simulink model "Alireza_3P_FuzzyPID"  (R2023a)
settings: Solver=VariableStepAuto  StartTime=0.0  StopTime=4  RelTol=1e-3
libraries: fuzblock x3, slpidlib x3
settings Model: Creator=Javad  LastModifiedBy=Alireza
settings SolverCC: AlgebraicLoopSolver=TrustRegion
settings DebuggingCC: UnconnectedInputMsg=warning  UnconnectedOutputMsg=warning  UnconnectedLineMsg=warning
settings ModelReferenceCC: EnableRefExpFcnMdlSchedulingChecks=on

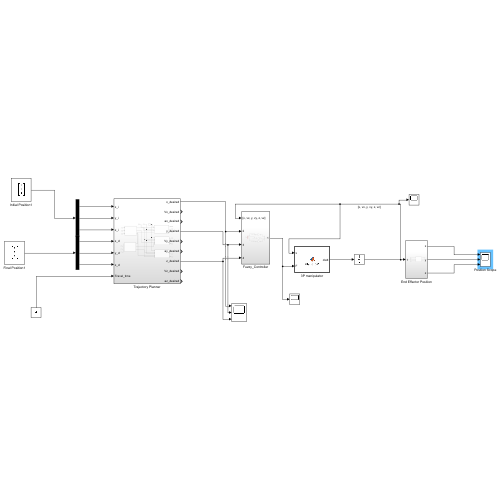
[thumbnail: Simulink's stored preview of the top-level diagram]
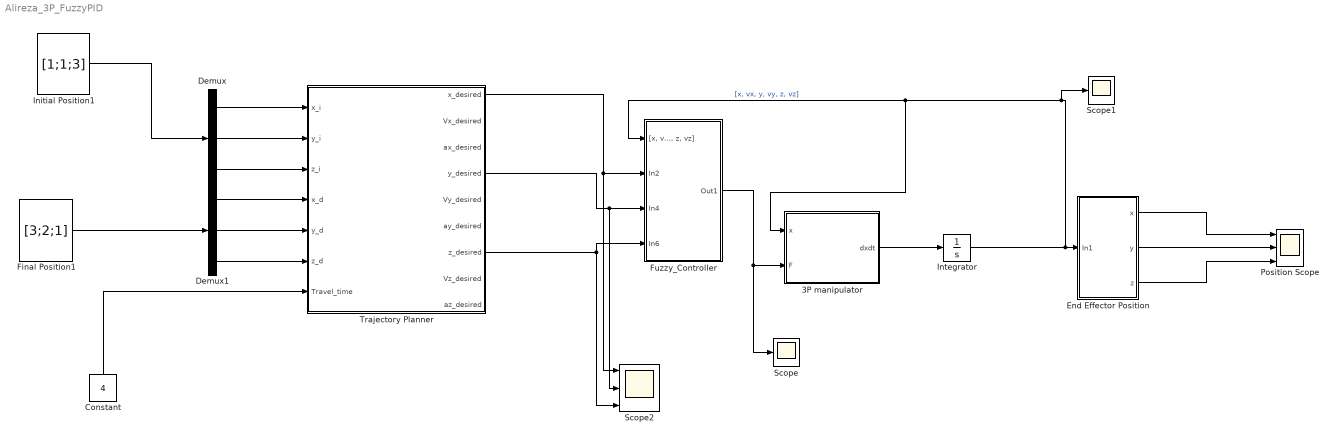
== system Alireza_3P_FuzzyPID ==
  3P manipulator : MATLAB Function  TreatAsAtomicUnit=on
  Constant : Constant  Value=4
  Demux : Demux  Outputs=3
  Demux1 : Demux  Outputs=3
  End Effector Position : Subsystem
  Final Position1 : Constant  Value=[3;2;1]  VectorParams1D=off
  Fuzzy_Controller : Subsystem
  Initial Position1 : Constant  Value=[1;1;3]  VectorParams1D=off
  Integrator : Integrator  InitialCondition=[0.5;0; 0.5;0; 2.8;0]
  Position Scope : Scope  NumInputPorts=3
  Scope : Scope
  Scope1 : Scope
  Scope2 : Scope  NumInputPorts=3
  Trajectory Planner : Subsystem
  wires:
  Demux/1 -> Trajectory Planner/1(x_i)
  Demux/2 -> Trajectory Planner/2(y_i)
  Demux/3 -> Trajectory Planner/3(z_i)
  Demux1/1 -> Trajectory Planner/4(x_d)
  Demux1/2 -> Trajectory Planner/5(y_d)
  Demux1/3 -> Trajectory Planner/6(z_d)
  3P manipulator/1(dxdt) -> Integrator/1
  Integrator/1 -> Scope1/1, 3P manipulator/1(x), Fuzzy_Controller/1("[x, vx, y, vy, z, vz]"), End Effector Position/1(In1)  "[x, vx, y, vy, z, vz]"
  End Effector Position/1(x) -> Position Scope/1
  End Effector Position/2(y) -> Position Scope/2
  End Effector Position/3(z) -> Position Scope/3
  Trajectory Planner/1(x_desired) -> Fuzzy_Controller/2(In2), Scope2/1
  Trajectory Planner/4(y_desired) -> Scope2/2, Fuzzy_Controller/3(In4)
  Trajectory Planner/7(z_desired) -> Fuzzy_Controller/4(In6), Scope2/3
  Fuzzy_Controller/1(Out1) -> Scope/1, 3P manipulator/2(F)
  Initial Position1/1 -> Demux/1
  Final Position1/1 -> Demux1/1
  Constant/1 -> Trajectory Planner/7(Travel_time)

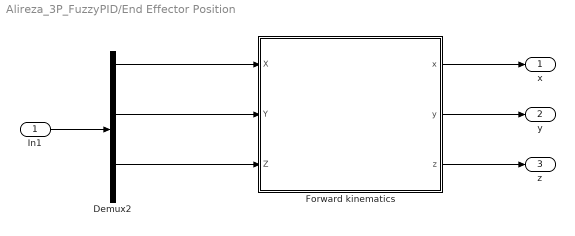
== system Alireza_3P_FuzzyPID/End Effector Position ==
  In1 : Inport
  Demux2 : Demux  Outputs=6
  Forward kinematics : MATLAB Function  TreatAsAtomicUnit=on
  x : Outport
  y : Outport  Port=2
  z : Outport  Port=3
  wires:
  Demux2/1 -> Forward kinematics/1(X)
  In1/1 -> Demux2/1
  Forward kinematics/2(y) -> y/1
  Demux2/3 -> Forward kinematics/2(Y)
  Forward kinematics/3(z) -> z/1
  Forward kinematics/1(x) -> x/1
  Demux2/5 -> Forward kinematics/3(Z)

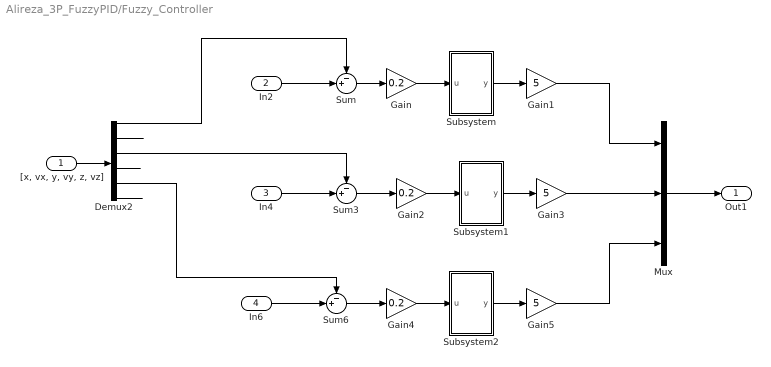
== system Alireza_3P_FuzzyPID/Fuzzy_Controller ==
  "[x, vx, y, vy, z, vz]" : Inport
  In2 : Inport  Port=2
  In4 : Inport  Port=3
  In6 : Inport  Port=4
  Demux2 : Demux  Outputs=6
  Gain : Gain  Gain=0.2
  Gain1 : Gain  Gain=5
  Gain2 : Gain  Gain=0.2
  Gain3 : Gain  Gain=5
  Gain4 : Gain  Gain=0.2
  Gain5 : Gain  Gain=5
  Mux : Mux  Inputs=3
  Subsystem : Subsystem
  Subsystem1 : Subsystem
  Subsystem2 : Subsystem
  Sum : Sum  Inputs=-+|
  Sum3 : Sum  Inputs=-+|
  Sum6 : Sum  Inputs=-+|
  Out1 : Outport
  wires:
  In2/1 -> Sum/2
  Demux2/5 -> Sum6/1
  In4/1 -> Sum3/2
  Demux2/1 -> Sum/1
  Demux2/2 -> ?
  Demux2/3 -> Sum3/1
  Mux/1 -> Out1/1
  In6/1 -> Sum6/2
  Demux2/4 -> ?
  Demux2/6 -> ?
  "[x, vx, y, vy, z, vz]"/1 -> Demux2/1
  Sum/1 -> Gain/1
  Gain/1 -> Subsystem/1(u)
  Subsystem/1(y) -> Gain1/1
  Gain1/1 -> Mux/1
  Subsystem1/1(y) -> Gain3/1
  Gain2/1 -> Subsystem1/1(u)
  Sum3/1 -> Gain2/1
  Gain3/1 -> Mux/2
  Gain5/1 -> Mux/3
  Gain4/1 -> Subsystem2/1(u)
  Subsystem2/1(y) -> Gain5/1
  Sum6/1 -> Gain4/1

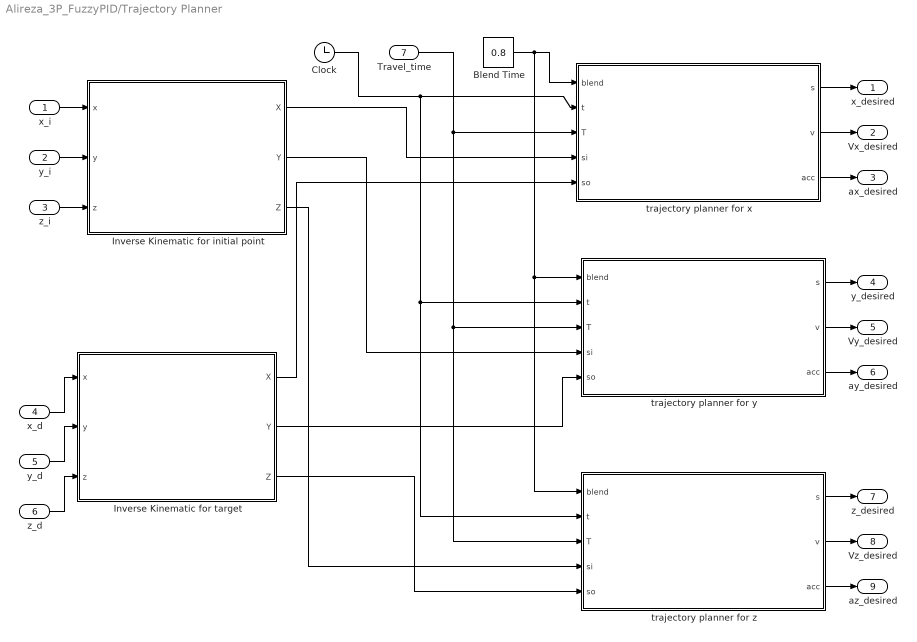
== system Alireza_3P_FuzzyPID/Trajectory Planner ==
  x_i : Inport
  y_i : Inport  Port=2
  z_i : Inport  Port=3
  x_d : Inport  Port=4
  y_d : Inport  Port=5
  z_d : Inport  Port=6
  Travel_time : Inport  Port=7
  Blend Time : Constant  Value=0.8
  Clock : Clock
  Inverse Kinematic for initial point : MATLAB Function  TreatAsAtomicUnit=on
  Inverse Kinematic for target : MATLAB Function  TreatAsAtomicUnit=on
  trajectory planner for x : MATLAB Function  TreatAsAtomicUnit=on
  trajectory planner for y : MATLAB Function  TreatAsAtomicUnit=on
  trajectory planner for z : MATLAB Function  TreatAsAtomicUnit=on
  x_desired : Outport
  Vx_desired : Outport  Port=2
  ax_desired : Outport  Port=3
  y_desired : Outport  Port=4
  Vy_desired : Outport  Port=5
  ay_desired : Outport  Port=6
  z_desired : Outport  Port=7
  Vz_desired : Outport  Port=8
  az_desired : Outport  Port=9
  wires:
  trajectory planner for x/2(v) -> Vx_desired/1
  y_i/1 -> Inverse Kinematic for initial point/2(y)
  trajectory planner for x/1(s) -> x_desired/1
  Inverse Kinematic for initial point/1(X) -> trajectory planner for x/4(si)
  Inverse Kinematic for target/1(X) -> trajectory planner for x/5(so)
  trajectory planner for x/3(acc) -> ax_desired/1
  x_i/1 -> Inverse Kinematic for initial point/1(x)
  z_i/1 -> Inverse Kinematic for initial point/3(z)
  Inverse Kinematic for initial point/2(Y) -> trajectory planner for y/4(si)
  trajectory planner for y/3(acc) -> ay_desired/1
  trajectory planner for y/2(v) -> Vy_desired/1
  trajectory planner for y/1(s) -> y_desired/1
  Inverse Kinematic for target/2(Y) -> trajectory planner for y/5(so)
  Clock/1 -> trajectory planner for x/2(t), trajectory planner for z/2(t), trajectory planner for y/2(t)
  Inverse Kinematic for target/3(Z) -> trajectory planner for z/5(so)
  trajectory planner for z/1(s) -> z_desired/1
  Inverse Kinematic for initial point/3(Z) -> trajectory planner for z/4(si)
  Travel_time/1 -> trajectory planner for x/3(T), trajectory planner for y/3(T), trajectory planner for z/3(T)
  trajectory planner for z/2(v) -> Vz_desired/1
  Blend Time/1 -> trajectory planner for y/1(blend), trajectory planner for z/1(blend), trajectory planner for x/1(blend)
  trajectory planner for z/3(acc) -> az_desired/1
  z_d/1 -> Inverse Kinematic for target/3(z)
  x_d/1 -> Inverse Kinematic for target/1(x)
  y_d/1 -> Inverse Kinematic for target/2(y)

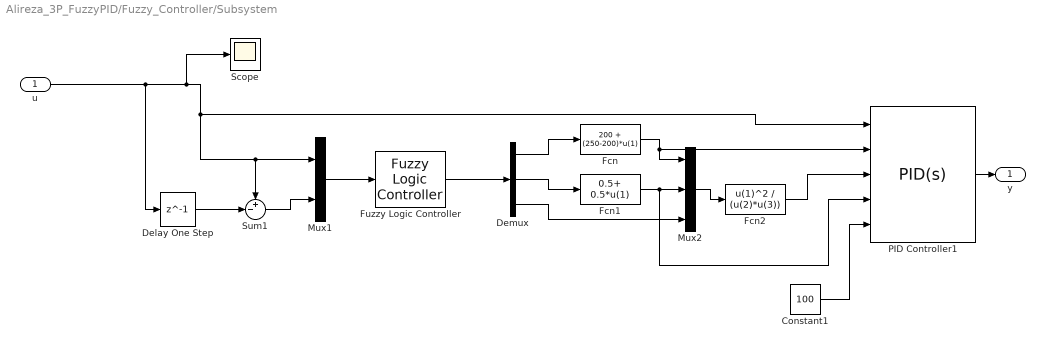
== system Alireza_3P_FuzzyPID/Fuzzy_Controller/Subsystem ==
  u : Inport
  Constant1 : Constant  Value=100
  Delay One Step : Delay  DelayLength=1
  Demux : Demux  Outputs=3
  Fcn : Fcn  Expr=200 + (250-200)*u(1)
  Fcn1 : Fcn  Expr=0.5+ 0.5*u(1)
  Fcn2 : Fcn  Expr=u(1)^2 / (u(2)*u(3))
  Fuzzy Logic Controller : fuzblock/Fuzzy Logic  Controller  FIS=fuzzy2  OutputSampleNumber=101  DataType=double  FuzzifiedInputs=off  RuleFiringStrengths=off  RuleOutputs=off  AggregatedOutputs=off  SimulateUsing=Code generation  OutOfRangeInputValueMessage=warning  NoRuleFiredMessage=warning  EmptyOutputFuzzySetMessage=warning
  Mux1 : Mux  Inputs=2
  Mux2 : Mux  Inputs=3
  PID Controller1 : slpidlib/PID Controller  Controller=PID  Form=Parallel  TimeDomain=Continuous-time  UseExternalTs=off  SampleTime=-1  IntegratorMethod=Forward Euler  FilterMethod=Forward Euler  ControllerParametersSource=external  P=4.74196748645127  I=1  UseKiTs=off  D=0  N=100  UseFilter=on  TunerSelectOption=Transfer Function Based (PID Tuner App)  InitialConditionSource=internal  InitialConditionForIntegrator=0  InitialConditionForFilter=0  DifferentiatorICPrevScaledInput=0  ExternalReset=none  TrackingMode=off  Kt=1  LimitOutput=off  SatLimitsSource=internal  UpperSaturationLimit=inf  LowerSaturationLimit=-inf  LinearizeAsGain=on  AntiWindupMode=none  Kb=1  LimitIntegrator=off  UpperIntegratorSaturationLimit=inf  LowerIntegratorSaturationLimit=-inf  POutMin=[]  POutMax=[]  IOutMin=[]  IOutMax=[]  DOutMin=[]  DOutMax=[]  NOutMin=[]  NOutMax=[]  SumOutMin=[]  SumOutMax=[]  SaturationOutMin=[]  SaturationOutMax=[]  PParamMin=[]  PParamMax=[]  IParamMin=[]  IParamMax=[]  DParamMin=[]  DParamMax=[]  NParamMin=[]  NParamMax=[]  KbParamMin=[]  KbParamMax=[]  KtParamMin=[]  KtParamMax=[]  KbOutMin=[]  KbOutMax=[]  KtOutMin=[]  KtOutMax=[]  IntegratorOutMin=[]  IntegratorOutMax=[]  FilterOutMin=[]  FilterOutMax=[]  SumI1OutMin=[]  SumI1OutMax=[]  SumI2OutMin=[]  SumI2OutMax=[]  SumI3OutMin=[]  SumI3OutMax=[]  SumI4OutMin=[]  SumI4OutMax=[]  SumDOutMin=[]  SumDOutMax=[]  DifferentiatorOutMin=[]  DifferentiatorOutMax=[]  FilterDiffOutCoefMin=[]  FilterDiffOutCoefMax=[]  ReciprocalOutMin=[]  ReciprocalOutMax=[]  SumDenOutMin=[]  SumDenOutMax=[]  SumNumOutMin=[]  SumNumOutMax=[]  DivideOutMin=[]  DivideOutMax=[]  UdiffTsProdOutMin=[]  UdiffTsProdOutMax=[]  NTsProdOutMin=[]  NTsProdOutMax=[]  UintegralTsProdOutMin=[]  UintegralTsProdOutMax=[]  UngainTsProdOutMin=[]  UngainTsProdOutMax=[]  ClampingZeroOutDataTypeStr=Inherit: Inherit via back propagation  ClampingZeroOutMin=[]  ClampingZeroOutMax=[]  FilterDenConstantOutDataTypeStr=Inherit: Inherit via back propagation  FilterDenConstantOutMin=[]  FilterDenConstantOutMax=[]  PCopyOutDataTypeStr=Inherit: Inherit via back propagation  PCopyOutMin=[]  PCopyOutMax=[]  NCopyOutDataTypeStr=Inherit: Inherit via back propagation  NCopyOutMin=[]  NCopyOutMax=[]  IntegratorContinuousStateAttributes=''  IntegratorStateMustResolveToSignalObject=off  IntegratorRTWStateStorageClass=Auto  FilterContinuousStateAttributes=''  FilterStateMustResolveToSignalObject=off  FilterRTWStateStorageClass=Auto  ParallelPVariant=ExternalParameters  IdealPVariant=Disabled  IVariant=ExternalParameters  DVariant=ExternalParameters  IntegratorVariant=Continuous  SatVariant=Disabled  AWVariant=Passthrough  PCopyVariant=Disabled  TRVariant=Disabled  FdbkBlocksVariant=Forward  IdealPFdbkVariant=Disabled  SatFdbkVariant=Disabled  DerivativeFilterVariant=ContFilter  NVariant=ExternalParameters  NCopyVariant=Disabled  FilterICVariant=InternalICsFilter  IntegratorICVariant=InternalICs  ExternalResetVariant=Disabled  TRSumVariant=Passthrough  SumFdbkVariant=Disabled  SumVariant=Sum_PID  TsampFilterVariant=InternalTs  TsampNgainVariant=Passthrough  TsampIntegralVariant=Disabled_SignalSpec  ExternalSaturationOutDataTypeStr=Inherit: Same as second input
  Scope : Scope
  Sum1 : Sum  Inputs=+-|
  y : Outport
  wires:
  Demux/1 -> Fcn/1
  Constant1/1 -> PID Controller1/5
  Mux1/1 -> Fuzzy Logic Controller/1
  Fuzzy Logic Controller/1 -> Demux/1
  Fcn/1 -> Mux2/1, PID Controller1/2
  Sum1/1 -> Mux1/2
  Delay One Step/1 -> Sum1/2
  Fcn2/1 -> PID Controller1/3
  Fcn1/1 -> PID Controller1/4, Mux2/2
  Mux2/1 -> Fcn2/1
  u/1 -> Delay One Step/1, Scope/1, Sum1/1, Mux1/1, PID Controller1/1
  Demux/2 -> Fcn1/1
  PID Controller1/1 -> y/1
  Demux/3 -> Mux2/3

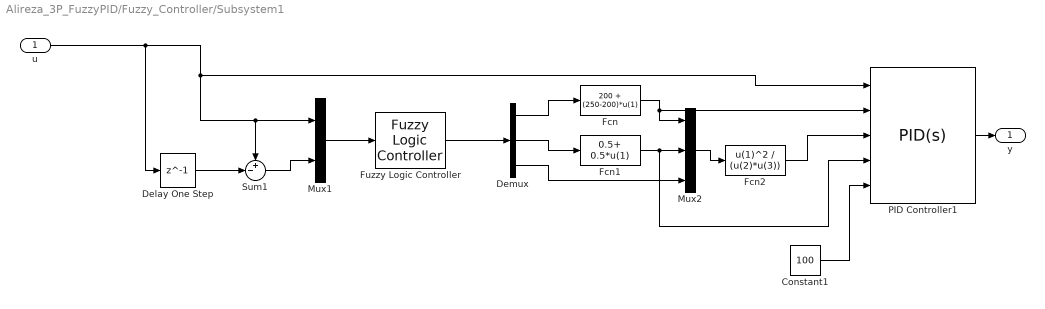
== system Alireza_3P_FuzzyPID/Fuzzy_Controller/Subsystem1 ==
  u : Inport
  Constant1 : Constant  Value=100
  Delay One Step : Delay  DelayLength=1
  Demux : Demux  Outputs=3
  Fcn : Fcn  Expr=200 + (250-200)*u(1)
  Fcn1 : Fcn  Expr=0.5+ 0.5*u(1)
  Fcn2 : Fcn  Expr=u(1)^2 / (u(2)*u(3))
  Fuzzy Logic Controller : fuzblock/Fuzzy Logic  Controller  FIS=fuzzy2  OutputSampleNumber=101  DataType=double  FuzzifiedInputs=off  RuleFiringStrengths=off  RuleOutputs=off  AggregatedOutputs=off  SimulateUsing=Code generation  OutOfRangeInputValueMessage=warning  NoRuleFiredMessage=warning  EmptyOutputFuzzySetMessage=warning
  Mux1 : Mux  Inputs=2
  Mux2 : Mux  Inputs=3
  PID Controller1 : slpidlib/PID Controller  Controller=PID  Form=Parallel  TimeDomain=Continuous-time  UseExternalTs=off  SampleTime=-1  IntegratorMethod=Forward Euler  FilterMethod=Forward Euler  ControllerParametersSource=external  P=4.74196748645127  I=1  UseKiTs=off  D=0  N=100  UseFilter=on  TunerSelectOption=Transfer Function Based (PID Tuner App)  InitialConditionSource=internal  InitialConditionForIntegrator=0  InitialConditionForFilter=0  DifferentiatorICPrevScaledInput=0  ExternalReset=none  TrackingMode=off  Kt=1  LimitOutput=off  SatLimitsSource=internal  UpperSaturationLimit=inf  LowerSaturationLimit=-inf  LinearizeAsGain=on  AntiWindupMode=none  Kb=1  LimitIntegrator=off  UpperIntegratorSaturationLimit=inf  LowerIntegratorSaturationLimit=-inf  POutMin=[]  POutMax=[]  IOutMin=[]  IOutMax=[]  DOutMin=[]  DOutMax=[]  NOutMin=[]  NOutMax=[]  SumOutMin=[]  SumOutMax=[]  SaturationOutMin=[]  SaturationOutMax=[]  PParamMin=[]  PParamMax=[]  IParamMin=[]  IParamMax=[]  DParamMin=[]  DParamMax=[]  NParamMin=[]  NParamMax=[]  KbParamMin=[]  KbParamMax=[]  KtParamMin=[]  KtParamMax=[]  KbOutMin=[]  KbOutMax=[]  KtOutMin=[]  KtOutMax=[]  IntegratorOutMin=[]  IntegratorOutMax=[]  FilterOutMin=[]  FilterOutMax=[]  SumI1OutMin=[]  SumI1OutMax=[]  SumI2OutMin=[]  SumI2OutMax=[]  SumI3OutMin=[]  SumI3OutMax=[]  SumI4OutMin=[]  SumI4OutMax=[]  SumDOutMin=[]  SumDOutMax=[]  DifferentiatorOutMin=[]  DifferentiatorOutMax=[]  FilterDiffOutCoefMin=[]  FilterDiffOutCoefMax=[]  ReciprocalOutMin=[]  ReciprocalOutMax=[]  SumDenOutMin=[]  SumDenOutMax=[]  SumNumOutMin=[]  SumNumOutMax=[]  DivideOutMin=[]  DivideOutMax=[]  UdiffTsProdOutMin=[]  UdiffTsProdOutMax=[]  NTsProdOutMin=[]  NTsProdOutMax=[]  UintegralTsProdOutMin=[]  UintegralTsProdOutMax=[]  UngainTsProdOutMin=[]  UngainTsProdOutMax=[]  ClampingZeroOutDataTypeStr=Inherit: Inherit via back propagation  ClampingZeroOutMin=[]  ClampingZeroOutMax=[]  FilterDenConstantOutDataTypeStr=Inherit: Inherit via back propagation  FilterDenConstantOutMin=[]  FilterDenConstantOutMax=[]  PCopyOutDataTypeStr=Inherit: Inherit via back propagation  PCopyOutMin=[]  PCopyOutMax=[]  NCopyOutDataTypeStr=Inherit: Inherit via back propagation  NCopyOutMin=[]  NCopyOutMax=[]  IntegratorContinuousStateAttributes=''  IntegratorStateMustResolveToSignalObject=off  IntegratorRTWStateStorageClass=Auto  FilterContinuousStateAttributes=''  FilterStateMustResolveToSignalObject=off  FilterRTWStateStorageClass=Auto  ParallelPVariant=ExternalParameters  IdealPVariant=Disabled  IVariant=ExternalParameters  DVariant=ExternalParameters  IntegratorVariant=Continuous  SatVariant=Disabled  AWVariant=Passthrough  PCopyVariant=Disabled  TRVariant=Disabled  FdbkBlocksVariant=Forward  IdealPFdbkVariant=Disabled  SatFdbkVariant=Disabled  DerivativeFilterVariant=ContFilter  NVariant=ExternalParameters  NCopyVariant=Disabled  FilterICVariant=InternalICsFilter  IntegratorICVariant=InternalICs  ExternalResetVariant=Disabled  TRSumVariant=Passthrough  SumFdbkVariant=Disabled  SumVariant=Sum_PID  TsampFilterVariant=InternalTs  TsampNgainVariant=Passthrough  TsampIntegralVariant=Disabled_SignalSpec  ExternalSaturationOutDataTypeStr=Inherit: Same as second input
  Sum1 : Sum  Inputs=+-|
  y : Outport
  wires:
  Demux/3 -> Mux2/3
  PID Controller1/1 -> y/1
  Demux/2 -> Fcn1/1
  u/1 -> PID Controller1/1, Mux1/1, Sum1/1, Delay One Step/1
  Mux2/1 -> Fcn2/1
  Fcn1/1 -> Mux2/2, PID Controller1/4
  Fcn2/1 -> PID Controller1/3
  Delay One Step/1 -> Sum1/2
  Sum1/1 -> Mux1/2
  Fcn/1 -> PID Controller1/2, Mux2/1
  Fuzzy Logic Controller/1 -> Demux/1
  Mux1/1 -> Fuzzy Logic Controller/1
  Constant1/1 -> PID Controller1/5
  Demux/1 -> Fcn/1

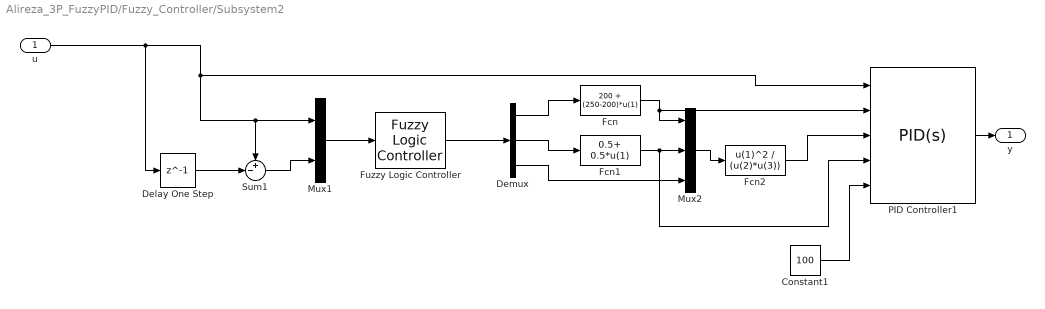
== system Alireza_3P_FuzzyPID/Fuzzy_Controller/Subsystem2 ==
  u : Inport
  Constant1 : Constant  Value=100
  Delay One Step : Delay  DelayLength=1
  Demux : Demux  Outputs=3
  Fcn : Fcn  Expr=200 + (250-200)*u(1)
  Fcn1 : Fcn  Expr=0.5+ 0.5*u(1)
  Fcn2 : Fcn  Expr=u(1)^2 / (u(2)*u(3))
  Fuzzy Logic Controller : fuzblock/Fuzzy Logic  Controller  FIS=fuzzy2  OutputSampleNumber=101  DataType=double  FuzzifiedInputs=off  RuleFiringStrengths=off  RuleOutputs=off  AggregatedOutputs=off  SimulateUsing=Code generation  OutOfRangeInputValueMessage=warning  NoRuleFiredMessage=warning  EmptyOutputFuzzySetMessage=warning
  Mux1 : Mux  Inputs=2
  Mux2 : Mux  Inputs=3
  PID Controller1 : slpidlib/PID Controller  Controller=PID  Form=Parallel  TimeDomain=Continuous-time  UseExternalTs=off  SampleTime=-1  IntegratorMethod=Forward Euler  FilterMethod=Forward Euler  ControllerParametersSource=external  P=4.74196748645127  I=1  UseKiTs=off  D=0  N=100  UseFilter=on  TunerSelectOption=Transfer Function Based (PID Tuner App)  InitialConditionSource=internal  InitialConditionForIntegrator=0  InitialConditionForFilter=0  DifferentiatorICPrevScaledInput=0  ExternalReset=none  TrackingMode=off  Kt=1  LimitOutput=off  SatLimitsSource=internal  UpperSaturationLimit=inf  LowerSaturationLimit=-inf  LinearizeAsGain=on  AntiWindupMode=none  Kb=1  LimitIntegrator=off  UpperIntegratorSaturationLimit=inf  LowerIntegratorSaturationLimit=-inf  POutMin=[]  POutMax=[]  IOutMin=[]  IOutMax=[]  DOutMin=[]  DOutMax=[]  NOutMin=[]  NOutMax=[]  SumOutMin=[]  SumOutMax=[]  SaturationOutMin=[]  SaturationOutMax=[]  PParamMin=[]  PParamMax=[]  IParamMin=[]  IParamMax=[]  DParamMin=[]  DParamMax=[]  NParamMin=[]  NParamMax=[]  KbParamMin=[]  KbParamMax=[]  KtParamMin=[]  KtParamMax=[]  KbOutMin=[]  KbOutMax=[]  KtOutMin=[]  KtOutMax=[]  IntegratorOutMin=[]  IntegratorOutMax=[]  FilterOutMin=[]  FilterOutMax=[]  SumI1OutMin=[]  SumI1OutMax=[]  SumI2OutMin=[]  SumI2OutMax=[]  SumI3OutMin=[]  SumI3OutMax=[]  SumI4OutMin=[]  SumI4OutMax=[]  SumDOutMin=[]  SumDOutMax=[]  DifferentiatorOutMin=[]  DifferentiatorOutMax=[]  FilterDiffOutCoefMin=[]  FilterDiffOutCoefMax=[]  ReciprocalOutMin=[]  ReciprocalOutMax=[]  SumDenOutMin=[]  SumDenOutMax=[]  SumNumOutMin=[]  SumNumOutMax=[]  DivideOutMin=[]  DivideOutMax=[]  UdiffTsProdOutMin=[]  UdiffTsProdOutMax=[]  NTsProdOutMin=[]  NTsProdOutMax=[]  UintegralTsProdOutMin=[]  UintegralTsProdOutMax=[]  UngainTsProdOutMin=[]  UngainTsProdOutMax=[]  ClampingZeroOutDataTypeStr=Inherit: Inherit via back propagation  ClampingZeroOutMin=[]  ClampingZeroOutMax=[]  FilterDenConstantOutDataTypeStr=Inherit: Inherit via back propagation  FilterDenConstantOutMin=[]  FilterDenConstantOutMax=[]  PCopyOutDataTypeStr=Inherit: Inherit via back propagation  PCopyOutMin=[]  PCopyOutMax=[]  NCopyOutDataTypeStr=Inherit: Inherit via back propagation  NCopyOutMin=[]  NCopyOutMax=[]  IntegratorContinuousStateAttributes=''  IntegratorStateMustResolveToSignalObject=off  IntegratorRTWStateStorageClass=Auto  FilterContinuousStateAttributes=''  FilterStateMustResolveToSignalObject=off  FilterRTWStateStorageClass=Auto  ParallelPVariant=ExternalParameters  IdealPVariant=Disabled  IVariant=ExternalParameters  DVariant=ExternalParameters  IntegratorVariant=Continuous  SatVariant=Disabled  AWVariant=Passthrough  PCopyVariant=Disabled  TRVariant=Disabled  FdbkBlocksVariant=Forward  IdealPFdbkVariant=Disabled  SatFdbkVariant=Disabled  DerivativeFilterVariant=ContFilter  NVariant=ExternalParameters  NCopyVariant=Disabled  FilterICVariant=InternalICsFilter  IntegratorICVariant=InternalICs  ExternalResetVariant=Disabled  TRSumVariant=Passthrough  SumFdbkVariant=Disabled  SumVariant=Sum_PID  TsampFilterVariant=InternalTs  TsampNgainVariant=Passthrough  TsampIntegralVariant=Disabled_SignalSpec  ExternalSaturationOutDataTypeStr=Inherit: Same as second input
  Sum1 : Sum  Inputs=+-|
  y : Outport
  wires:
  Demux/1 -> Fcn/1
  Constant1/1 -> PID Controller1/5
  Mux1/1 -> Fuzzy Logic Controller/1
  Fuzzy Logic Controller/1 -> Demux/1
  Fcn/1 -> Mux2/1, PID Controller1/2
  Sum1/1 -> Mux1/2
  Delay One Step/1 -> Sum1/2
  Fcn2/1 -> PID Controller1/3
  Fcn1/1 -> PID Controller1/4, Mux2/2
  Mux2/1 -> Fcn2/1
  u/1 -> Delay One Step/1, Sum1/1, Mux1/1, PID Controller1/1
  Demux/2 -> Fcn1/1
  PID Controller1/1 -> y/1
  Demux/3 -> Mux2/3

== matlab function Alireza_3P_FuzzyPID/Trajectory Planner/Inverse Kinematic for initial point ==
  data: x input; X output; y input; z input; Y output; Z output
function [X, Y, Z] = inverse_kinematic(x, y, z)

L1=0.5; L2=0.5; L3=0.2;
X=x-L1;
Y=y-L2;
Z=z-L3;

end

== matlab function Alireza_3P_FuzzyPID/3P manipulator ==
  data: x input size=[6,1]; dxdt output size=[6,1]; F input size=[3,1]

function dxdt = Plant_3P (x, F)
m1 = 15; m2 = 10; m3 = 5; M =1; g=9.8;
dxdt = zeros(6,1);
dxdt(1) = x(2);
dxdt(2) = 1/(m2+m3+M)*(F(1));
dxdt(3) = x(4);
dxdt(4) = 1/(m1+m2+m3+M)*(F(2));
dxdt(5) = x(6);
dxdt(6) = 1/(M+m3)*(-(M+m3)*g+F(3));

end

== matlab function Alireza_3P_FuzzyPID/Trajectory Planner/trajectory planner for x ==
  data: blend input; t input; s output; T input; si input; so input; v output; acc output
function [s, v, acc] = trajectory_planner(blend, t, T, si, so)
%t is the current time
%T is the toal time of the movement. 
%si is the initial position
%so is the target position
% blend = 1;

V_max = (so-si)/(T-blend);
a = V_max/blend;

if t<=blend
    acc = a;
    v = a*t;
    s = 1/2*a*t.^2+si;
elseif t<=(T-blend)
    acc = 0;
    v = V_max;
    s = 1/2*a*blend^2+si+V_max.*(t-blend);
else
    acc = -a;
    v = V_max-a.*(t-(T-blend));
    s = -1/2*a.*(t-(T-blend)).^2+V_max*(t-(T-blend))+1/2*a*blend^2+si+...
        V_max*(T-2*blend);
end
    
end

== matlab function Alireza_3P_FuzzyPID/Trajectory Planner/trajectory planner for y ==
  data: blend input; t input; s output; T input; si input; so input; v output; acc output
function [s, v, acc] = trajectory_planner(blend, t, T, si, so)
%t is the current time
%T is the toal time of the movement. 
%si is the initial position
%so is the target position
% blend = 1;

V_max = (so-si)/(T-blend);
a = V_max/blend;

if t<=blend
    acc = a;
    v = a*t;
    s = 1/2*a*t.^2+si;
elseif t<=(T-blend)
    acc = 0;
    v = V_max;
    s = 1/2*a*blend^2+si+V_max.*(t-blend);
else
    acc = -a;
    v = V_max-a.*(t-(T-blend));
    s = -1/2*a.*(t-(T-blend)).^2+V_max*(t-(T-blend))+1/2*a*blend^2+si+...
        V_max*(T-2*blend);
end
    
end

== matlab function Alireza_3P_FuzzyPID/Trajectory Planner/trajectory planner for z ==
  data: blend input; t input; s output; T input; si input; so input; v output; acc output
function [s, v, acc] = trajectory_planner(blend, t, T, si, so)
%t is the current time
%T is the toal time of the movement. 
%si is the initial position
%so is the target position
% blend = 1;

V_max = (so-si)/(T-blend);
a = V_max/blend;

if t<=blend
    acc = a;
    v = a*t;
    s = 1/2*a*t.^2+si;
elseif t<=(T-blend)
    acc = 0;
    v = V_max;
    s = 1/2*a*blend^2+si+V_max.*(t-blend);
else
    acc = -a;
    v = V_max-a.*(t-(T-blend));
    s = -1/2*a.*(t-(T-blend)).^2+V_max*(t-(T-blend))+1/2*a*blend^2+si+...
        V_max*(T-2*blend);
end
    
end

== matlab function Alireza_3P_FuzzyPID/Trajectory Planner/Inverse Kinematic for target ==
  data: x input; X output; y input; z input; Y output; Z output
function [X, Y, Z] = inverse_kinematic(x, y, z)

L1=0.5; L2=0.5; L3=0.2;
X=x-L1;
Y=y-L2;
Z=z-L3;

end

== matlab function Alireza_3P_FuzzyPID/End Effector Position/Forward kinematics ==
  data: x output; X input; y output; Y input; Z input; z output
function [x, y, z] = fcn(X, Y, Z)
L1=0.5; L2=0.5; L3=0.2;
x=X+L1;
y=Y+L2;
z=Z+L3;

end
